simulink model "Child-Phone-MS"  (R2023a)
settings: Solver=FixedStepAuto  StartTime=0.0  StopTime=inf  RelTol=1e-3
undefined symbols (not defined in the file): altitud, Danger_level, finalcs0x2810x29, lati, long
libraries: androidaudiovideolib x4, androiduilib x4, androidcommunicationlib x4, androidsensorlib x3, fuzblock x1
settings Model: Creator=ketha  LastModifiedBy=ketha
settings OptimizationCC: EnhancedBackFolding=on  PassReuseOutputArgsAs=Individual arguments  ZeroExternalMemoryAtStartup=off  ZeroInternalMemoryAtStartup=off  MaxStackSize=64  OptimizeBlockOrder=speed  DifferentSizesBufferReuse=on  OptimizationCustomize=off  EfficientTunableParamExpr=on
settings DebuggingCC: ParameterTunabilityLossMsg=error
settings HardwareCC: ProdBitPerPointer=32  ProdBitPerSizeT=32  ProdBitPerPtrDiffT=32  ProdLargestAtomicInteger=Long  ProdLargestAtomicFloat=Double  ProdWordSize=32  ProdHWDeviceType=ARM Compatible->ARM Cortex  UseEmbeddedCoderFeatures=off
settings SFSimCC: MATLABDynamicMemAlloc=off
settings RTWCC: Description=Embedded Coder  SystemTargetFile=ert.tlc  HardwareBoard=Android Device  TLCOptions="-aInlineSetEventsForThisBaseRateFcn=TLC_FALSE -aSuppressMultiTaskScheduler=TLC_FALSE  -aRateBasedStepFcn=0"  TemplateMakefile=ert_default_tmf  RTWVerbose=off  Toolchain=Android SDK/NDK Tools
settings CodeAppCC: ForceParamTrailComments=on  IgnoreCustomStorageClasses=off  OperatorAnnotations=on  SimulinkDataObjDesc=on  SFDataObjDesc=on  InsertBlockDesc=on
settings ERTTargetCC: SupportContinuousTime=on  SupportNonInlinedSFcns=on

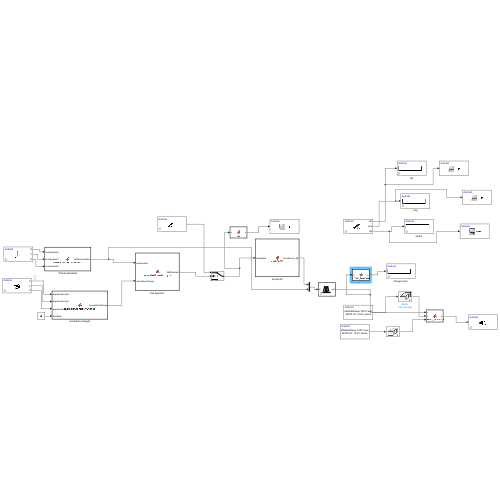
[thumbnail: Simulink's stored preview of the top-level diagram]
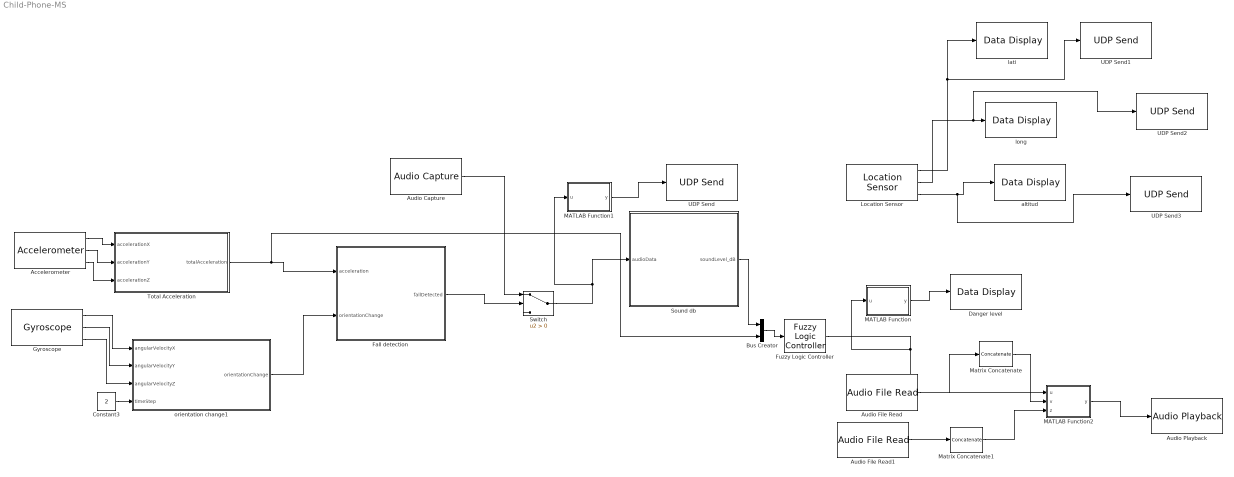
== system Child-Phone-MS ==
  Accelerometer : androidsensorlib/Accelerometer  OutputVector=off  SampleTime=0.1  BlockPlatform=Android
  Audio Capture : androidaudiovideolib/Audio Capture  SampleFreq=44100  FrameSize=4410  SampleTime=0.1  SimulateUsing=Code generation  DeviceStr=0  QueueDuration=0  BlockPlatform=Android  AudioSamplingFreq=44100
  Audio File Read : androidaudiovideolib/Audio File Read  FileName=C:\Users\ketha\Downloads\attack2t22wav-14511.wav  FrameSize=2400
  Audio File Read1 : androidaudiovideolib/Audio File Read  FileName=C:\Users\ketha\Downloads\attack2t22wav-14511.wav  FrameSize=2400
  Audio Playback : androidaudiovideolib/Audio Playback  SampleFreq=24000  AudioSamplingFreq=24000  SampleTime=0.1  DeviceStr=0  QueueDuration=0  BlockPlatform=Android
  Bus Creator : BusCreator  Inputs=2
  Constant3 : Constant  Value=2
  Danger level : androiduilib/Data Display  DataDisplayId=finalcs0x2810x29/Danger_level  Format=Float  Precision=6  SimulateUsing=Code generation  blockPlatform=Android
  Fall detection : MATLAB Function  TreatAsAtomicUnit=on
  Fuzzy Logic Controller : fuzblock/Fuzzy Logic  Controller  FIS=fuzzy_logic  OutputSampleNumber=101  DataType=double  FuzzifiedInputs=off  RuleFiringStrengths=off  RuleOutputs=off  AggregatedOutputs=off  SimulateUsing=Interpreted execution  OutOfRangeInputValueMessage=warning  NoRuleFiredMessage=warning  EmptyOutputFuzzySetMessage=warning
  Gyroscope : androidsensorlib/Gyroscope  OutputVector=off  SampleTime=0.1  BlockPlatform=Android
  Location Sensor : androidsensorlib/Location Sensor  OutputVector=off  SampleTime=0.1  BlockPlatform=Android
  MATLAB Function : MATLAB Function  TreatAsAtomicUnit=on
  MATLAB Function1 : MATLAB Function  TreatAsAtomicUnit=on
  MATLAB Function2 : MATLAB Function  TreatAsAtomicUnit=on
  Matrix Concatenate : Concatenate  NumInputs=1  Mode=Multidimensional array  ConcatenateDimension=2
  Matrix Concatenate1 : Concatenate  NumInputs=1  Mode=Multidimensional array  ConcatenateDimension=2
  Sound db : MATLAB Function  TreatAsAtomicUnit=on
  Switch : Switch  Criteria=u2 > Threshold  SaturateOnIntegerOverflow=off  InputSameDT=off
  Total Acceleration : MATLAB Function  TreatAsAtomicUnit=on
  UDP Send : androidcommunicationlib/UDP Send  remoteURL='10.7.52.92'  remotePort=32000  localURL='0.0.0.0'  localPortSource=Automatically determine  localPort=-1  sampletime=-1  blockPlatform=Android  separateLengthPort=0
  UDP Send1 : androidcommunicationlib/UDP Send  remoteURL='10.7.52.92'  remotePort=25000  localURL='0.0.0.0'  localPortSource=Automatically determine  localPort=-1  sampletime=-1  blockPlatform=Android  separateLengthPort=0
  UDP Send2 : androidcommunicationlib/UDP Send  remoteURL='10.7.52.92'  remotePort=26000  localURL='0.0.0.0'  localPortSource=Automatically determine  localPort=-1  sampletime=-1  blockPlatform=Android  separateLengthPort=0
  UDP Send3 : androidcommunicationlib/UDP Send  remoteURL='10.7.52.92'  remotePort=27000  localURL='0.0.0.0'  localPortSource=Automatically determine  localPort=-1  sampletime=-1  blockPlatform=Android  separateLengthPort=0
  altitud : androiduilib/Data Display  DataDisplayId=finalcs0x2810x29/altitud  Format=Float  Precision=6  SimulateUsing=Code generation  blockPlatform=Android
  lati : androiduilib/Data Display  DataDisplayId=finalcs0x2810x29/lati  Format=Float  Precision=6  SimulateUsing=Code generation  blockPlatform=Android
  long : androiduilib/Data Display  DataDisplayId=finalcs0x2810x29/long  Format=Float  Precision=6  SimulateUsing=Code generation  blockPlatform=Android
  orientation change1 : MATLAB Function  TreatAsAtomicUnit=on
  wires:
  Constant3/1 -> orientation change1/4(timeStep)
  Gyroscope/3 -> orientation change1/3(angularVelocityZ)
  Gyroscope/2 -> orientation change1/2(angularVelocityY)
  Gyroscope/1 -> orientation change1/1(angularVelocityX)
  Accelerometer/2 -> Total Acceleration/2(accelerationY)
  Accelerometer/3 -> Total Acceleration/3(accelerationZ)
  Accelerometer/1 -> Total Acceleration/1(accelerationX)
  orientation change1/1(orientationChange) -> Fall detection/2(orientationChange)
  Fuzzy Logic Controller/1 -> MATLAB Function2/1(u), MATLAB Function/1(u)
  MATLAB Function/1(y) -> Danger level/1
  MATLAB Function1/1(y) -> UDP Send/1
  Audio File Read/1 -> Matrix Concatenate/1
  Audio File Read1/1 -> Matrix Concatenate1/1
  Matrix Concatenate/1 -> MATLAB Function2/2(v)
  Matrix Concatenate1/1 -> MATLAB Function2/3(z)
  MATLAB Function2/1(y) -> Audio Playback/1
  Total Acceleration/1(totalAcceleration) -> Bus Creator/2, Fall detection/1(acceleration)
  Fall detection/1(fallDetected) -> Switch/2
  Audio Capture/1 -> Switch/1
  Switch/1 -> MATLAB Function1/1(u), Sound db/1(audioData)
  Sound db/1(soundLevel_dB) -> Bus Creator/1
  Bus Creator/1 -> Fuzzy Logic Controller/1
  Location Sensor/1 -> lati/1, UDP Send1/1
  Location Sensor/2 -> UDP Send2/1, long/1
  Location Sensor/3 -> UDP Send3/1, altitud/1

== matlab function Child-Phone-MS/orientation change1 ==
  data: angularVelocityX input; orientationChange output; angularVelocityY input; angularVelocityZ input; timeStep input
function orientationChange = calculateOrientationChange(angularVelocityX, angularVelocityY, angularVelocityZ, timeStep)
    persistent orientation
    
    if isempty(orientation)
        orientation = single([0; 0; 0]); % Initial orientation as single precision
    end
    
    % Integrate angular velocities to obtain orientation change
    pitch = single(angularVelocityX * timeStep); % Ensure single precision
    roll = single(angularVelocityY * timeStep); % Ensure single precision
    yaw = single(angularVelocityZ * timeStep);   % Ensure single precision
    
    % Update orientation
    orientation = orientation + single([pitch; roll; yaw]); % Ensure single precision
    
    % Calculate total orientation change (sum of pitch, roll, and yaw)
    orientationChange = sum(orientation);
    
 
end

== matlab function Child-Phone-MS/Total Acceleration ==
  data: accelerationX input; totalAcceleration output; accelerationY input; accelerationZ input
function totalAcceleration = calculateTotalAcceleration(accelerationX, accelerationY, accelerationZ)
    % Calculate total acceleration magnitude using Euclidean norm
    totalAcceleration = sqrt(accelerationX.^2 + accelerationY.^2 + accelerationZ.^2);
end

== matlab function Child-Phone-MS/MATLAB Function1 ==
  data: u input; y output
function y = fcn(u)

y = u(:);

== matlab function Child-Phone-MS/MATLAB Function2 ==
  data: u input; y output; v input; z input
function y = output_selection(u,v,z)
   
    if u >= 7 && u <= 10
        y =v*0,1;
    else
        y = z*0;
    end
end

== matlab function Child-Phone-MS/Fall detection ==
  data: acceleration input; fallDetected output; orientationChange input
function fallDetected = detectFallFromMotorcycle(acceleration, orientationChange)
    % Thresholds for fall detection
    decelerationThreshold = -10; % Threshold for abrupt deceleration (m/s^2)
    impactThreshold = 30; % Threshold for impact (m/s^2)
    maxorientationChangeThreshold = 30; % Threshold for orientation change (degrees)
    minorientationchangethreshold=-25;


    % Initialize fall detection result
    fallDetected = 0;

    % Case 1: Abrupt deceleration
    if min(acceleration) < decelerationThreshold
        fallDetected = 1;
        return;
    end


    % Case 3: Impact
    if max(abs(acceleration)) > impactThreshold
        fallDetected = 1;
        return;
    end

    % Case 5: Orientation change
    if (orientationChange) > maxorientationChangeThreshold
        fallDetected = 1;
        return;
    end
     if (orientationChange) <minorientationchangethreshold
        fallDetected = 1;
        return;
     end
end

== matlab function Child-Phone-MS/MATLAB Function ==
  data: u input; y output
function y = output_selection(u)
    if u < 7
        y = 1;
    elseif u >= 7 && u <= 8
        y = 2;
    else
        y = 3;
    end
end

== matlab function Child-Phone-MS/Sound db ==
  data: audioData input; soundLevel_dB output
function soundLevel_dB = audioToDB(audioData)
    % Calculate sound level in dB
    % Assuming audioData is the captured audio signal
    
    % Calculate the RMS (root mean square) values of each channel of the audio data
    rmsValue = rms(audioData, 1); % Compute RMS along each column (dimension 1)
    
    % Calculate the average RMS value across all channels
    avgRMS = mean(rmsValue);
    
    % Perform the calculation in double precision
    dblResult = 20 * log10(avgRMS);
    
    % Cast the result to single precision
    soundLevel_dB = single(dblResult);
end
